simulink library "nort_sysgenlib"  (Simulink 6.5)
undefined symbols (not defined in the file or in its folder): Down, Up
libraries: xbsIndex_r4 x338, nort_sysgenlib x10
(part 1 of 2)
settings Model: Creator=nort  LastModifiedBy=nort

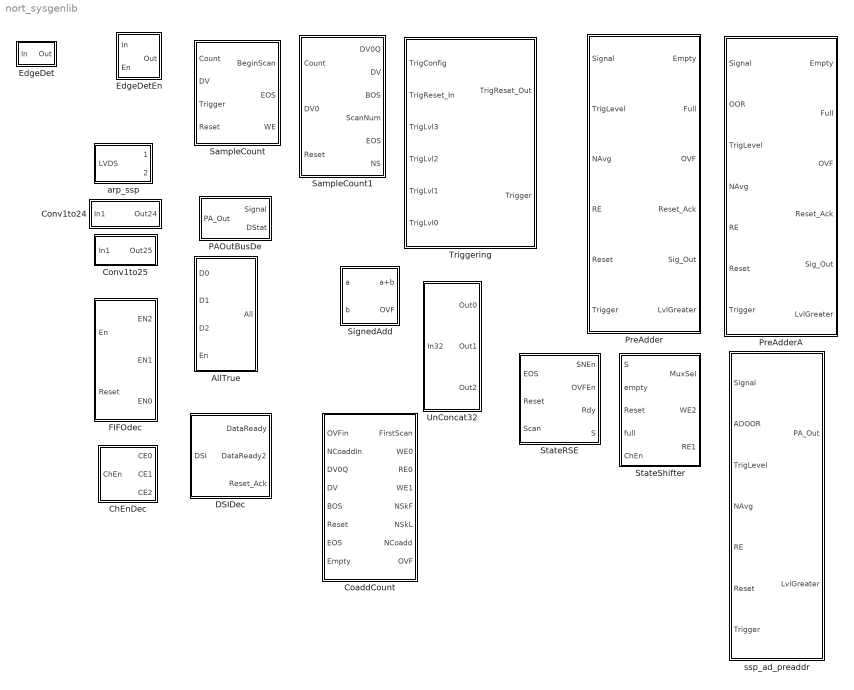
== system nort_sysgenlib ==
  AllTrue : Subsystem
  ChEnDec : Subsystem
  CoaddCount : Subsystem
  Conv1to24 : Subsystem
  Conv1to25 : Subsystem
  DSIDec : Subsystem
  EdgeDet : Subsystem
  EdgeDetEn : Subsystem
  FIFOdec : Subsystem
  PAOutBusDe : Subsystem
  PreAdder : Subsystem
  PreAdderA : Subsystem
  SampleCount : Subsystem
  SampleCount1 : Subsystem
  SignedAdd : Subsystem
  StateRSE : Subsystem
  StateShifter : Subsystem
  Triggering : Subsystem
  UnConcat32 : Subsystem
  arp_ssp : Subsystem
  ssp_ad_preaddr : Subsystem

== system nort_sysgenlib/AllTrue ==
  note: AllTrue: March 7, 2008
  note: Output is true if all
      | the enabled inputs
      | are true.
  D0 : Inport
  D1 : Inport  Port=2
  D2 : Inport  Port=3
  En : Inport  Port=4
  ChEnDec : nort_sysgenlib/ChEnDec  SystemSampleTime=-1
  Inverter : xbsIndex_r4/Inverter  en=off  latency=0  dbl_ovrd=off  block_type=inv
      settings: block_version=9.2.01
  Inverter1 : xbsIndex_r4/Inverter  en=off  latency=0  dbl_ovrd=off  block_type=inv
      settings: block_version=9.2.01
  Inverter2 : xbsIndex_r4/Inverter  en=off  latency=0  dbl_ovrd=off  block_type=inv
      settings: block_version=9.2.01
  Logical1 : xbsIndex_r4/Logical  logical_function=OR  inputs=2  en=off  latency=0  precision=Full  arith_type=Unsigned  n_bits=16  bin_pt=0  align_bp=on  dbl_ovrd=off  block_type=logical
      settings: block_version=9.2.01
  Logical2 : xbsIndex_r4/Logical  logical_function=AND  inputs=3  en=off  latency=0  precision=Full  arith_type=Unsigned  n_bits=16  bin_pt=0  align_bp=on  dbl_ovrd=off  block_type=logical
      settings: block_version=9.2.01
  Logical4 : xbsIndex_r4/Logical  logical_function=OR  inputs=2  en=off  latency=0  precision=Full  arith_type=Unsigned  n_bits=16  bin_pt=0  align_bp=on  dbl_ovrd=off  block_type=logical
      settings: block_version=9.2.01
  Logical6 : xbsIndex_r4/Logical  logical_function=OR  inputs=2  en=off  latency=0  precision=Full  arith_type=Unsigned  n_bits=16  bin_pt=0  align_bp=on  dbl_ovrd=off  block_type=logical
      settings: block_version=9.2.01
  All : Outport
  wires:
  En/1 -> ChEnDec/1
  ChEnDec/3 -> Inverter2/1
  ChEnDec/2 -> Inverter1/1
  ChEnDec/1 -> Inverter/1
  D2/1 -> Logical6/1
  Logical2/1 -> All/1
  D1/1 -> Logical4/1
  D0/1 -> Logical1/1
  Logical6/1 -> Logical2/3
  Logical1/1 -> Logical2/1
  Logical4/1 -> Logical2/2
  Inverter/1 -> Logical1/2
  Inverter1/1 -> Logical4/2
  Inverter2/1 -> Logical6/2

== system nort_sysgenlib/ChEnDec ==
  note: ChEnDec: March 7, 2008
  ChEn : Inport
  ChEnblBit0 : xbsIndex_r4/Slice  nbits=3  boolean_output=on  mode=Lower Bit Location + Width  bit1=0  base1=MSB of Input  bit0=0  base0=LSB of Input  dbl_ovrd=off  block_type=slice
      settings: infoedit="Extracts a given range of bits from each input sample and presents it at the output.  The output type is ordinarily unsigned with binary point at zero, but can be Boolean when the slice is one bit wide.<P><P>Hardware notes: In hardware this block costs nothing."  block_version=8.2
  ChEnblBit1 : xbsIndex_r4/Slice  nbits=3  boolean_output=on  mode=Lower Bit Location + Width  bit1=0  base1=MSB of Input  bit0=1  base0=LSB of Input  dbl_ovrd=off  block_type=slice
      settings: infoedit="Extracts a given range of bits from each input sample and presents it at the output.  The output type is ordinarily unsigned with binary point at zero, but can be Boolean when the slice is one bit wide.<P><P>Hardware notes: In hardware this block costs nothing."  block_version=8.2
  ChEnblBit2 : xbsIndex_r4/Slice  nbits=3  boolean_output=on  mode=Lower Bit Location + Width  bit1=0  base1=MSB of Input  bit0=2  base0=LSB of Input  dbl_ovrd=off  block_type=slice
      settings: infoedit="Extracts a given range of bits from each input sample and presents it at the output.  The output type is ordinarily unsigned with binary point at zero, but can be Boolean when the slice is one bit wide.<P><P>Hardware notes: In hardware this block costs nothing."  block_version=8.2
  CE0 : Outport
  CE1 : Outport  Port=2
  CE2 : Outport  Port=3
  wires:
  ChEnblBit2/1 -> CE2/1
  ChEnblBit1/1 -> CE1/1
  ChEnblBit0/1 -> CE0/1
  ChEn/1 -> ChEnblBit2/1, ChEnblBit1/1, ChEnblBit0/1

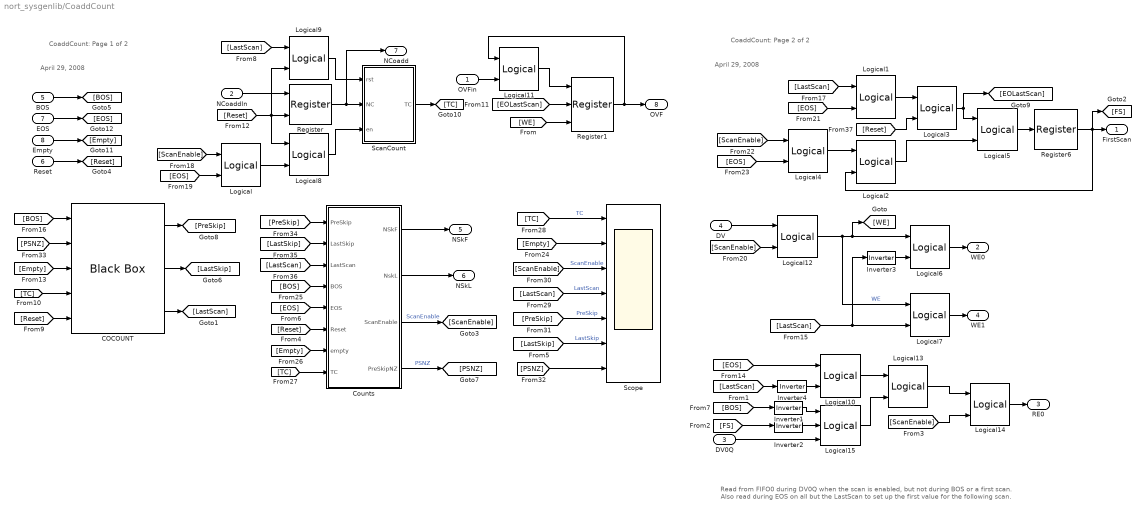
== system nort_sysgenlib/CoaddCount ==
  note: Read from FIFO0 during DV0Q when the scan is enabled, but not during BOS or a first scan.
      | Also read during EOS on all but the LastScan to set up the first value for the following scan.
  note: April 29, 2008
  note: CoaddCount: Page 2 of 2
  note: April 29, 2008
  note: CoaddCount: Page 1 of 2
  OVFin : Inport
  NCoaddIn : Inport  Port=2
  DV0Q : Inport  Port=3
  DV : Inport  Port=4
  BOS : Inport  Port=5
  Reset : Inport  Port=6
  EOS : Inport  Port=7
  Empty : Inport  Port=8
  COCOUNT : xbsIndex_r4/Black Box  init_code=COCOUNT_config  sim_method=ISE Simulator  block_type=blackbox2
      settings: infoedit="Incorporates black box HDL and simulation model into a System Generator design.<P><P>You must supply a Black Box with certain information about the HDL component you would like to bring into System Generator. This information is provided through a Matlab function.<P><P>When \"Simulation mode\" is set to \"Inactive\", you will typically want to provide a separate simulation model by using a Simulation Multiplexer.<P>When \"Simulation mode\" is set to \"External co-simulator\", you must include a ModelSim block in the design."  block_version=9.2.01
  Counts : Subsystem
  Inverter{1..4} (4 alike) : xbsIndex_r4/Inverter  en=off  latency=0  dbl_ovrd=off  block_type=inv
      settings: block_version=9.2.01
  Logical{,1..2,6..7,10,12,14} (8 alike) : xbsIndex_r4/Logical  logical_function=AND  inputs=2  en=off  latency=0  precision=Full  arith_type=Unsigned  n_bits=16  bin_pt=0  align_bp=on  dbl_ovrd=off  block_type=logical
      settings: block_version=9.2.01
  Logical{3,5,8..9,11,13} (6 alike) : xbsIndex_r4/Logical  logical_function=OR  inputs=2  en=off  latency=0  precision=Full  arith_type=Unsigned  n_bits=16  bin_pt=0  align_bp=on  dbl_ovrd=off  block_type=logical
      settings: block_version=9.2.01
  Logical15 : xbsIndex_r4/Logical  logical_function=AND  inputs=3  en=off  latency=0  precision=Full  arith_type=Unsigned  n_bits=16  bin_pt=0  align_bp=on  dbl_ovrd=off  block_type=logical
      settings: block_version=9.2.01
  Logical4 : xbsIndex_r4/Logical  logical_function=NAND  inputs=2  en=off  latency=0  precision=Full  arith_type=Unsigned  n_bits=16  bin_pt=0  align_bp=on  dbl_ovrd=off  block_type=logical
      settings: block_version=9.2.01
  Register : xbsIndex_r4/Register  init=0  rst=off  en=on  dbl_ovrd=off  block_type=register
      settings: block_version=9.2.01
  Register1 : xbsIndex_r4/Register  init=0  rst=on  en=on  dbl_ovrd=off  block_type=register
      settings: block_version=9.2.01
  Register6 : xbsIndex_r4/Register  init=0  rst=off  en=off  dbl_ovrd=off  block_type=register
      settings: block_version=9.2.01
  ScanCount : Subsystem
  Scope : Scope  NumInputPorts=7
      settings: TickLabels=on  TimeRange=5000  YMin=-0.25~-0.25~-0.15~-0.25~-0.25~-0.25~-0.25  YMax=1.25~1.25~1.25~1.25~1.25~1.25~1.25
  FirstScan : Outport
  WE0 : Outport  Port=2
  RE0 : Outport  Port=3
  WE1 : Outport  Port=4
  NSkF : Outport  Port=5
  NSkL : Outport  Port=6
  NCoadd : Outport  Port=7
  OVF : Outport  Port=8
  wires:
  Logical3/1 -> [EOLastScan], Logical5/1
  Logical5/1 -> Register6/1
  Inverter2/1 -> Logical15/2
  Inverter1/1 -> Logical15/1
  [Reset] -> Logical3/2
  [LastScan] -> Counts/3(LastScan)
  [LastSkip] -> Counts/2(LastSkip)
  [PreSkip] -> Counts/1(PreSkip)
  [PSNZ] -> COCOUNT/2
  [PSNZ] -> Scope/7
  [TC] -> Counts/8(TC)
  [Empty] -> Counts/7(empty)
  [BOS] -> Counts/4(BOS)
  COCOUNT/2 -> [LastSkip]
  COCOUNT/3 -> [LastScan]
  [Empty] -> Scope/2
  [ScanEnable] -> Logical14/2
  [EOS] -> Logical4/2
  [ScanEnable] -> Logical4/1
  Logical4/1 -> Logical2/1
  Logical2/1 -> Logical5/2
  Logical1/1 -> Logical3/1
  [EOS] -> Logical1/2
  [LastScan] -> Logical1/1
  [EOS] -> Logical/2
  [ScanEnable] -> Logical/1
  Counts/4(PreSkipNZ) -> [PSNZ]  "PSNZ"
  [BOS] -> COCOUNT/1
  [Empty] -> COCOUNT/3
  [TC] -> COCOUNT/4
  [Reset] -> COCOUNT/5
  [LastScan] -> Logical9/1
  EOS/1 -> [EOS]
  [LastSkip] -> Scope/6  "LastSkip"
  [PreSkip] -> Scope/5  "PreSkip"
  [ScanEnable] -> Scope/3  "ScanEnable"
  [LastScan] -> Scope/4  "LastScan"
  [TC] -> Scope/1  "TC"
  Logical14/1 -> RE0/1
  Logical15/1 -> Logical13/2
  [FS] -> Inverter2/1
  Inverter4/1 -> Logical10/2
  Logical10/1 -> Logical13/1
  DV0Q/1 -> Logical15/3
  Logical13/1 -> Logical14/1
  [LastScan] -> Inverter4/1
  Logical11/1 -> Register1/1
  [WE] -> Register1/3
  Logical12/1 -> Logical7/1, Logical6/1, [WE]  "WE"
  Register1/1 -> Logical11/1, OVF/1
  OVFin/1 -> Logical11/2
  Logical9/1 -> ScanCount/1(rst)
  Logical8/1 -> ScanCount/3(en)
  Logical7/1 -> WE1/1
  Logical6/1 -> WE0/1
  Inverter3/1 -> Logical6/2
  DV/1 -> Logical12/1
  Counts/3(ScanEnable) -> [ScanEnable]  "ScanEnable"
  COCOUNT/1 -> [PreSkip]
  BOS/1 -> [BOS]
  Empty/1 -> [Empty]
  ScanCount/1(TC) -> [TC]
  Register6/1 -> Logical2/2, [FS], FirstScan/1
  Counts/2(NskL) -> NSkL/1
  Counts/1(NSkF) -> NSkF/1
  Register/1 -> NCoadd/1, ScanCount/2(NC)
  NCoaddIn/1 -> Register/1
  Reset/1 -> [Reset]
  [Reset] -> Counts/6(Reset)
  [EOS] -> Counts/5(EOS)
  [BOS] -> Inverter1/1
  [EOLastScan] -> Register1/2
  [Reset] -> Logical8/1, Register/2, Logical9/2
  Logical/1 -> Logical8/2
  [EOS] -> Logical10/1
  [LastScan] -> Logical7/2, Inverter3/1
  [ScanEnable] -> Logical12/2

== system nort_sysgenlib/Conv1to24 ==
  In1 : Inport
  To24Bits : xbsIndex_r4/Convert  arith_type="Signed  (2's comp)"  n_bits=24  bin_pt=0  quantization=Truncate  overflow=Wrap  latency=0  dbl_ovrd=off  pipeline=off  block_type=convert
      settings: block_version=9.2.01
  ToSigned : xbsIndex_r4/Convert  arith_type="Signed  (2's comp)"  n_bits=1  bin_pt=0  quantization=Truncate  overflow=Wrap  latency=0  dbl_ovrd=off  pipeline=off  block_type=convert
      settings: block_version=9.2.01
  Out24 : Outport
  wires:
  In1/1 -> ToSigned/1
  ToSigned/1 -> To24Bits/1
  To24Bits/1 -> Out24/1

== system nort_sysgenlib/Conv1to25 ==
  In1 : Inport
  To25Bits : xbsIndex_r4/Convert  arith_type="Signed  (2's comp)"  n_bits=25  bin_pt=0  quantization=Truncate  overflow=Wrap  latency=0  dbl_ovrd=off  pipeline=off  block_type=convert
      settings: block_version=9.2.01
  ToSigned : xbsIndex_r4/Convert  arith_type="Signed  (2's comp)"  n_bits=1  bin_pt=0  quantization=Truncate  overflow=Wrap  latency=0  dbl_ovrd=off  pipeline=off  block_type=convert
      settings: block_version=9.2.01
  Out25 : Outport
  wires:
  In1/1 -> ToSigned/1
  ToSigned/1 -> To25Bits/1
  To25Bits/1 -> Out25/1

== system nort_sysgenlib/DSIDec ==
  note: DSIDec: April 29, 2008
  DSI : Inport
  Empty_Bit2 : xbsIndex_r4/Slice  nbits=1  boolean_output=on  mode=Lower Bit Location + Width  bit1=0  base1=MSB of Input  bit0=2  base0=LSB of Input  dbl_ovrd=off  block_type=slice
      settings: infoedit="Extracts a given range of bits from each input sample and presents it at the output.  The output type is ordinarily unsigned with binary point at zero, but can be Boolean when the slice is one bit wide.<P><P>Hardware notes: In hardware this block costs nothing."  block_version=9.2.01
  Full_Bit1 : xbsIndex_r4/Slice  nbits=1  boolean_output=on  mode=Lower Bit Location + Width  bit1=0  base1=MSB of Input  bit0=1  base0=LSB of Input  dbl_ovrd=off  block_type=slice
      settings: infoedit="Extracts a given range of bits from each input sample and presents it at the output.  The output type is ordinarily unsigned with binary point at zero, but can be Boolean when the slice is one bit wide.<P><P>Hardware notes: In hardware this block costs nothing."  block_version=9.2.01
  Inverter2 : xbsIndex_r4/Inverter  en=off  latency=0  dbl_ovrd=off  block_type=inv
      settings: block_version=9.2.01
  RAck_Bit0 : xbsIndex_r4/Slice  nbits=1  boolean_output=on  mode=Lower Bit Location + Width  bit1=0  base1=MSB of Input  bit0=0  base0=LSB of Input  dbl_ovrd=off  block_type=slice
      settings: infoedit="Extracts a given range of bits from each input sample and presents it at the output.  The output type is ordinarily unsigned with binary point at zero, but can be Boolean when the slice is one bit wide.<P><P>Hardware notes: In hardware this block costs nothing."  block_version=9.2.01
  DataReady : Outport
  DataReady2 : Outport  Port=2
  Reset_Ack : Outport  Port=3
  wires:
  RAck_Bit0/1 -> Reset_Ack/1
  Full_Bit1/1 -> DataReady2/1
  Inverter2/1 -> DataReady/1
  Empty_Bit2/1 -> Inverter2/1
  DSI/1 -> RAck_Bit0/1, Full_Bit1/1, Empty_Bit2/1

== system nort_sysgenlib/EdgeDet ==
  note: Simple Edge Detector
  In : Inport
  Delay : xbsIndex_r4/Delay  en=off  latency=1  dbl_ovrd=off  reg_retiming=off  block_type=delay
      settings: block_version=9.1.01
  Delay1 : xbsIndex_r4/Delay  en=off  latency=1  dbl_ovrd=off  reg_retiming=off  block_type=delay
      settings: block_version=9.1.01
  Inverter1 : xbsIndex_r4/Inverter  en=off  latency=0  dbl_ovrd=off  block_type=inv
      settings: block_version=9.1.01
  Logical3 : xbsIndex_r4/Logical  logical_function=AND  inputs=2  en=off  latency=0  precision=Full  arith_type=Unsigned  n_bits=16  bin_pt=0  align_bp=on  dbl_ovrd=off  block_type=logical
      settings: block_version=9.1.01
  Out : Outport
  wires:
  Delay1/1 -> Delay/1, Logical3/2
  Logical3/1 -> Out/1
  Inverter1/1 -> Logical3/1
  Delay/1 -> Inverter1/1
  In/1 -> Delay1/1

== system nort_sysgenlib/EdgeDetEn ==
  note: Edge Detection with Enable
  In : Inport
  En : Inport  Port=2
  Delay : xbsIndex_r4/Delay  en=off  latency=1  dbl_ovrd=off  reg_retiming=off  block_type=delay
      settings: block_version=9.1.01
  Delay1 : xbsIndex_r4/Delay  en=on  latency=1  dbl_ovrd=off  reg_retiming=off  block_type=delay
      settings: block_version=9.1.01
  Inverter1 : xbsIndex_r4/Inverter  en=off  latency=0  dbl_ovrd=off  block_type=inv
      settings: block_version=9.1.01
  Logical3 : xbsIndex_r4/Logical  logical_function=AND  inputs=2  en=off  latency=0  precision=Full  arith_type=Unsigned  n_bits=16  bin_pt=0  align_bp=on  dbl_ovrd=off  block_type=logical
      settings: block_version=9.1.01
  Out : Outport
  wires:
  En/1 -> Delay1/2
  In/1 -> Delay1/1
  Delay1/1 -> Delay/1, Logical3/2
  Logical3/1 -> Out/1
  Inverter1/1 -> Logical3/1
  Delay/1 -> Inverter1/1

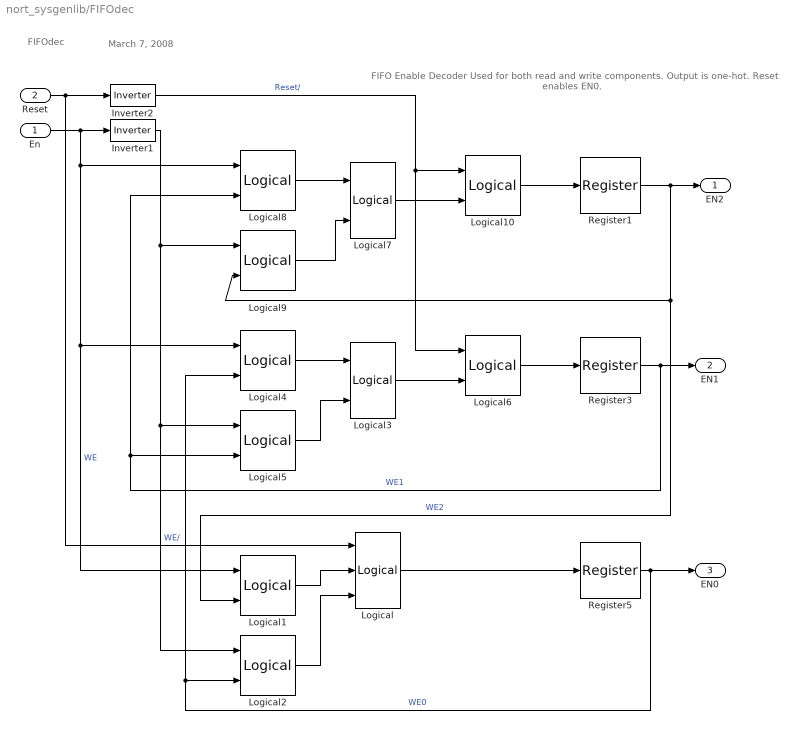
== system nort_sysgenlib/FIFOdec ==
  note: FIFO Enable Decoder
      | Used for both read and write components.
      | Output is one-hot. Reset enables EN0.
  note: March 7, 2008
  note: FIFOdec
  En : Inport
  Reset : Inport  Port=2
  Inverter1 : xbsIndex_r4/Inverter  en=off  latency=0  dbl_ovrd=off  block_type=inv
      settings: block_version=9.2.01
  Inverter2 : xbsIndex_r4/Inverter  en=off  latency=0  dbl_ovrd=off  block_type=inv
      settings: block_version=9.2.01
  Logical : xbsIndex_r4/Logical  logical_function=OR  inputs=3  en=off  latency=0  precision=Full  arith_type=Unsigned  n_bits=16  bin_pt=0  align_bp=on  dbl_ovrd=off  block_type=logical
      settings: block_version=9.2.01
  Logical{1..2,4..6,8..10} (8 alike) : xbsIndex_r4/Logical  logical_function=AND  inputs=2  en=off  latency=0  precision=Full  arith_type=Unsigned  n_bits=16  bin_pt=0  align_bp=on  dbl_ovrd=off  block_type=logical
      settings: block_version=9.2.01
  Logical3 : xbsIndex_r4/Logical  logical_function=OR  inputs=2  en=off  latency=0  precision=Full  arith_type=Unsigned  n_bits=16  bin_pt=0  align_bp=on  dbl_ovrd=off  block_type=logical
      settings: block_version=9.2.01
  Logical7 : xbsIndex_r4/Logical  logical_function=OR  inputs=2  en=off  latency=0  precision=Full  arith_type=Unsigned  n_bits=16  bin_pt=0  align_bp=on  dbl_ovrd=off  block_type=logical
      settings: block_version=9.2.01
  Register1 : xbsIndex_r4/Register  init=0  rst=off  en=off  dbl_ovrd=off  block_type=register
      settings: block_version=9.2.01
  Register3 : xbsIndex_r4/Register  init=0  rst=off  en=off  dbl_ovrd=off  block_type=register
      settings: block_version=9.2.01
  Register5 : xbsIndex_r4/Register  init=0  rst=off  en=off  dbl_ovrd=off  block_type=register
      settings: block_version=9.2.01
  EN2 : Outport
  EN1 : Outport  Port=2
  EN0 : Outport  Port=3
  wires:
  Logical8/1 -> Logical7/1
  Inverter2/1 -> Logical10/1, Logical6/1  "Reset/"
  Logical10/1 -> Register1/1
  Logical7/1 -> Logical10/2
  Logical9/1 -> Logical7/2
  Logical6/1 -> Register3/1
  Logical3/1 -> Logical6/2
  Logical4/1 -> Logical3/1
  Logical5/1 -> Logical3/2
  Logical1/1 -> Logical/2
  Logical2/1 -> Logical/3
  Inverter1/1 -> Logical9/1, Logical5/1, Logical2/1  "WE/"
  En/1 -> Logical8/1, Logical4/1, Logical1/1, Inverter1/1  "WE"
  Reset/1 -> Inverter2/1, Logical/1
  Logical/1 -> Register5/1
  Register5/1 -> Logical4/2, Logical2/2, EN0/1  "WE0"
  Register3/1 -> Logical8/2, Logical5/2, EN1/1  "WE1"
  Register1/1 -> Logical9/2, Logical1/2, EN2/1  "WE2"

== system nort_sysgenlib/PAOutBusDe ==
  note: PAOutBusDecode: April 29, 2008
  PA_Out : Inport
  DS_Bot3 : xbsIndex_r4/Slice  nbits=3  boolean_output=off  mode=Lower Bit Location + Width  bit1=0  base1=MSB of Input  bit0=0  base0=LSB of Input  dbl_ovrd=off  block_type=slice
      settings: infoedit="Extracts a given range of bits from each input sample and presents it at the output.  The output type is ordinarily unsigned with binary point at zero, but can be Boolean when the slice is one bit wide.<P><P>Hardware notes: In hardware this block costs nothing."  block_version=9.2.01
  Sig_Top26 : xbsIndex_r4/Slice  nbits=26  boolean_output=off  mode=Lower Bit Location + Width  bit1=0  base1=MSB of Input  bit0=3  base0=LSB of Input  dbl_ovrd=off  block_type=slice
      settings: infoedit="Extracts a given range of bits from each input sample and presents it at the output.  The output type is ordinarily unsigned with binary point at zero, but can be Boolean when the slice is one bit wide.<P><P>Hardware notes: In hardware this block costs nothing."  block_version=9.2.01
  Signal : Outport
  DStat : Outport  Port=2
  wires:
  DS_Bot3/1 -> DStat/1
  Sig_Top26/1 -> Signal/1
  PA_Out/1 -> Sig_Top26/1, DS_Bot3/1

== system nort_sysgenlib/PreAdder ==
  note: February 29, 2008
  note: ssp_ad_preaddr V2.00a
  Signal : Inport
  TrigLevel : Inport  Port=2
  NAvg : Inport  Port=3
  RE : Inport  Port=4
  Reset : Inport  Port=5
  Trigger : Inport  Port=6
  AddSub : xbsIndex_r4/AddSub  mode=Addition  use_carryin=off  use_carryout=off  en=off  latency=0  precision=User Defined  arith_type="Signed  (2's comp)"  n_bits=24  bin_pt=0  quantization=Truncate  overflow=Saturate  dbl_ovrd=off  use_behavioral_HDL=off  pipelined=off  use_rpm=on  block_type=addsub
      settings: block_version=9.1.01
  Count : Subsystem
  FIFO : Subsystem
  Logical : xbsIndex_r4/Logical  logical_function=OR  inputs=2  en=off  latency=0  precision=Full  arith_type=Unsigned  n_bits=16  bin_pt=0  align_bp=on  dbl_ovrd=off  block_type=logical
      settings: block_version=9.2.01
  Register : xbsIndex_r4/Register  init=0  rst=on  en=off  dbl_ovrd=off  block_type=register
      settings: block_version=9.1.01
  Relational : xbsIndex_r4/Relational  mode=a>b  en=off  latency=0  dbl_ovrd=off  block_type=relational
      settings: block_version=9.2.01
  State : Subsystem
  Empty : Outport
  Full : Outport  Port=2
  OVF : Outport  Port=3
  Reset_Ack : Outport  Port=4
  Sig_Out : Outport  Port=5
  LvlGreater : Outport  Port=6
  wires:
  FIFO/3(Full) -> Full/1  "Full"
  State/1(Inactive) -> Logical/2, Count/2(Reset)
  FIFO/4(OVF) -> OVF/1  "OVF"
  Trigger/1 -> State/2(Trigger)
  FIFO/2(Empty) -> Empty/1  "Empty"
  Reset/1 -> State/1(ResIn)
  NAvg/1 -> Count/1(NA)
  TrigLevel/1 -> Relational/2
  Relational/1 -> LvlGreater/1
  RE/1 -> FIFO/3(RE)
  Count/1(NewData) -> FIFO/2(WE), Logical/1  "NewData"
  Logical/1 -> Register/2
  State/2(Reset) -> Reset_Ack/1, FIFO/4(Reset)
  FIFO/1(Dout) -> Sig_Out/1  "Sig_Out"
  Signal/1 -> AddSub/2, Relational/1
  Register/1 -> AddSub/1
  AddSub/1 -> FIFO/1(Din), Register/1

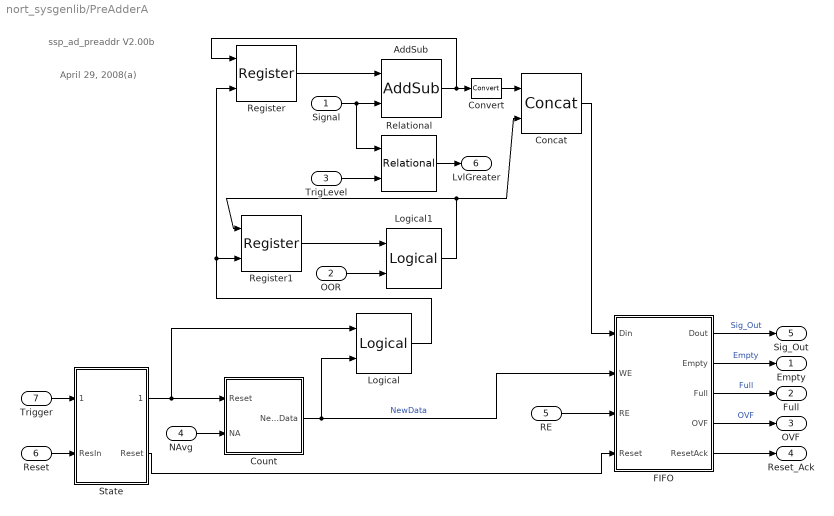
== system nort_sysgenlib/PreAdderA ==
  note: April 29, 2008(a)
  note: ssp_ad_preaddr V2.00b
  Signal : Inport
  OOR : Inport  Port=2
  TrigLevel : Inport  Port=3
  NAvg : Inport  Port=4
  RE : Inport  Port=5
  Reset : Inport  Port=6
  Trigger : Inport  Port=7
  AddSub : xbsIndex_r4/AddSub  mode=Addition  use_carryin=off  use_carryout=off  en=off  latency=0  precision=User Defined  arith_type="Signed  (2's comp)"  n_bits=24  bin_pt=0  quantization=Truncate  overflow=Saturate  dbl_ovrd=off  use_behavioral_HDL=off  pipelined=off  use_rpm=on  block_type=addsub
      settings: block_version=9.1.01
  Concat : xbsIndex_r4/Concat  num_inputs=2  dbl_ovrd=off  block_type=concat
      settings: block_version=9.2.01
  Convert : xbsIndex_r4/Convert  arith_type=Unsigned  n_bits=24  bin_pt=0  quantization=Truncate  overflow=Wrap  latency=0  dbl_ovrd=off  pipeline=off  block_type=convert
      settings: block_version=9.2.01
  Count : Subsystem
  FIFO : Subsystem
  Logical : xbsIndex_r4/Logical  logical_function=OR  inputs=2  en=off  latency=0  precision=Full  arith_type=Unsigned  n_bits=16  bin_pt=0  align_bp=on  dbl_ovrd=off  block_type=logical
      settings: block_version=9.2.01
  Logical1 : xbsIndex_r4/Logical  logical_function=OR  inputs=2  en=off  latency=0  precision=Full  arith_type=Unsigned  n_bits=16  bin_pt=0  align_bp=on  dbl_ovrd=off  block_type=logical
      settings: block_version=9.2.01
  Register : xbsIndex_r4/Register  init=0  rst=on  en=off  dbl_ovrd=off  block_type=register
      settings: block_version=9.1.01
  Register1 : xbsIndex_r4/Register  init=0  rst=on  en=off  dbl_ovrd=off  block_type=register
      settings: block_version=9.1.01
  Relational : xbsIndex_r4/Relational  mode=a>b  en=off  latency=0  dbl_ovrd=off  block_type=relational
      settings: block_version=9.2.01
  State : Subsystem
  Empty : Outport
  Full : Outport  Port=2
  OVF : Outport  Port=3
  Reset_Ack : Outport  Port=4
  Sig_Out : Outport  Port=5
  LvlGreater : Outport  Port=6
  wires:
  Logical/1 -> Register1/2, Register/2
  FIFO/5(ResetAck) -> Reset_Ack/1
  Convert/1 -> Concat/1
  FIFO/3(Full) -> Full/1  "Full"
  State/1(Inactive) -> Logical/1, Count/1(Reset)
  FIFO/4(OVF) -> OVF/1  "OVF"
  Trigger/1 -> State/1(Trigger)
  FIFO/2(Empty) -> Empty/1  "Empty"
  Reset/1 -> State/2(ResIn)
  NAvg/1 -> Count/2(NA)
  TrigLevel/1 -> Relational/2
  Relational/1 -> LvlGreater/1
  RE/1 -> FIFO/3(RE)
  Count/1(NewData) -> Logical/2, FIFO/2(WE)  "NewData"
  State/2(Reset) -> FIFO/4(Reset)
  FIFO/1(Dout) -> Sig_Out/1  "Sig_Out"
  Signal/1 -> AddSub/2, Relational/1
  Register/1 -> AddSub/1
  AddSub/1 -> Convert/1, Register/1
  Logical1/1 -> Concat/2, Register1/1
  Register1/1 -> Logical1/1
  OOR/1 -> Logical1/2
  Concat/1 -> FIFO/1(Din)

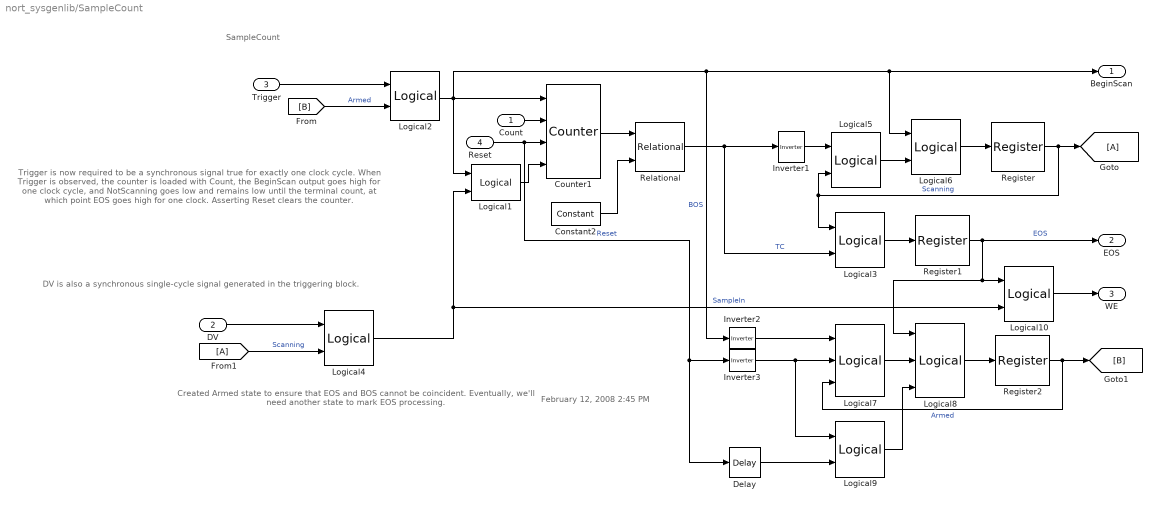
== system nort_sysgenlib/SampleCount ==
  note: Trigger is now required to be a
      | synchronous signal true for exactly
      | one clock cycle. When Trigger
      | is observed, the counter is loaded
      | with Count, the BeginScan output goes
      | high for one clock cycle, and
      | NotScanning goes low and remains low
      | until the terminal count, at which point
      | EOS goes high for one clock.
      | Asserting Reset clears the counter.
  note: February 12, 2008 2:45 PM
  note: DV is also a synchronous single-cycle signal
      | generated in the triggering block.
  note: SampleCount
  note: Created Armed state to ensure that EOS and BOS cannot be coincident.
      | Eventually, we'll need another state to mark EOS processing.
  Count : Inport
  DV : Inport  Port=2
  Trigger : Inport  Port=3
  Reset : Inport  Port=4
  Constant2 : xbsIndex_r4/Constant  arith_type=Unsigned  const=0  n_bits=11  bin_pt=0  explicit_period=off  period=1  equ=P=C  opselect=C  inp2=PCIN>>17  opr=+  inp1=P  carry=CIN  dbl_ovrd=off  block_type=constant
      settings: block_version=8.2
  Counter1 : xbsIndex_r4/Counter  cnt_type=Free Running  cnt_to=Inf  operation=Down  start_count=0  cnt_by_val=1  arith_type=Unsigned  n_bits=12  bin_pt=0  load_pin=on  rst=on  en=on  explicit_period=off  period=1  dbl_ovrd=off  use_behavioral_HDL=off  use_rpm=off  block_type=counter
      settings: block_version=8.2
  Delay : xbsIndex_r4/Delay  en=off  latency=1  dbl_ovrd=off  reg_retiming=off  block_type=delay
      settings: block_version=9.2.01
  Inverter1 : xbsIndex_r4/Inverter  en=off  latency=0  dbl_ovrd=off  block_type=inv
      settings: block_version=8.2
  Inverter2 : xbsIndex_r4/Inverter  en=off  latency=0  dbl_ovrd=off  block_type=inv
      settings: block_version=8.2
  Inverter3 : xbsIndex_r4/Inverter  en=off  latency=0  dbl_ovrd=off  block_type=inv
      settings: block_version=8.2
  Logical1 : xbsIndex_r4/Logical  logical_function=OR  inputs=2  en=off  latency=0  precision=Full  arith_type=Unsigned  n_bits=16  bin_pt=0  align_bp=on  dbl_ovrd=off  block_type=logical
      settings: block_version=8.2
  Logical10 : xbsIndex_r4/Logical  logical_function=OR  inputs=2  en=off  latency=0  precision=Full  arith_type=Unsigned  n_bits=1  bin_pt=0  align_bp=off  dbl_ovrd=off  block_type=logical
      settings: block_version=8.2
  Logical2 : xbsIndex_r4/Logical  logical_function=AND  inputs=2  en=off  latency=0  precision=Full  arith_type=Unsigned  n_bits=16  bin_pt=0  align_bp=on  dbl_ovrd=off  block_type=logical
      settings: block_version=8.2
  Logical{3..5,9} (4 alike) : xbsIndex_r4/Logical  logical_function=AND  inputs=2  en=off  latency=0  precision=Full  arith_type=Unsigned  n_bits=1  bin_pt=0  align_bp=off  dbl_ovrd=off  block_type=logical
      settings: block_version=8.2
  Logical6 : xbsIndex_r4/Logical  logical_function=OR  inputs=2  en=off  latency=0  precision=Full  arith_type=Unsigned  n_bits=1  bin_pt=0  align_bp=off  dbl_ovrd=off  block_type=logical
      settings: block_version=8.2
  Logical7 : xbsIndex_r4/Logical  logical_function=AND  inputs=3  en=off  latency=0  precision=Full  arith_type=Unsigned  n_bits=1  bin_pt=0  align_bp=off  dbl_ovrd=off  block_type=logical
      settings: block_version=8.2
  Logical8 : xbsIndex_r4/Logical  logical_function=OR  inputs=3  en=off  latency=0  precision=Full  arith_type=Unsigned  n_bits=1  bin_pt=0  align_bp=off  dbl_ovrd=off  block_type=logical
      settings: block_version=8.2
  Register : xbsIndex_r4/Register  init=0  rst=off  en=off  dbl_ovrd=off  block_type=register
      settings: block_version=9.2.01
  Register1 : xbsIndex_r4/Register  init=0  rst=off  en=off  dbl_ovrd=off  block_type=register
      settings: block_version=9.2.01
  Register2 : xbsIndex_r4/Register  init=0  rst=off  en=off  dbl_ovrd=off  block_type=register
      settings: block_version=9.2.01
  Relational : xbsIndex_r4/Relational  mode=a=b  en=off  latency=0  dbl_ovrd=off  block_type=relational
      settings: block_version=8.2
  BeginScan : Outport
  EOS : Outport  Port=2
  WE : Outport  Port=3
  wires:
  Counter1/1 -> Relational/1
  Logical1/1 -> Counter1/4
  Constant2/1 -> Relational/2
  Logical2/1 -> Counter1/1, Logical1/1, BeginScan/1, Logical6/1, Inverter2/1  "BOS"
  Count/1 -> Counter1/2
  Trigger/1 -> Logical2/1
  Reset/1 -> Counter1/3, Delay/1, Inverter3/1  "Reset"
  Logical4/1 -> Logical10/2, Logical1/2  "SampleIn"
  [A] -> Logical4/2  "Scanning"
  DV/1 -> Logical4/1
  Logical5/1 -> Logical6/2
  Logical6/1 -> Register/1
  Inverter1/1 -> Logical5/1
  Relational/1 -> Logical3/2, Inverter1/1  "TC"
  Register/1 -> Logical5/2, Logical3/1, [A]  "Scanning"
  Logical3/1 -> Register1/1
  Register1/1 -> EOS/1, Logical8/1, Logical10/1  "EOS"
  Inverter2/1 -> Logical7/1
  Logical8/1 -> Register2/1
  Logical7/1 -> Logical8/2
  Register2/1 -> Logical7/3, [B]  "Armed"
  [B] -> Logical2/2  "Armed"
  Inverter3/1 -> Logical7/2, Logical9/1
  Delay/1 -> Logical9/2
  Logical9/1 -> Logical8/3
  Logical10/1 -> WE/1

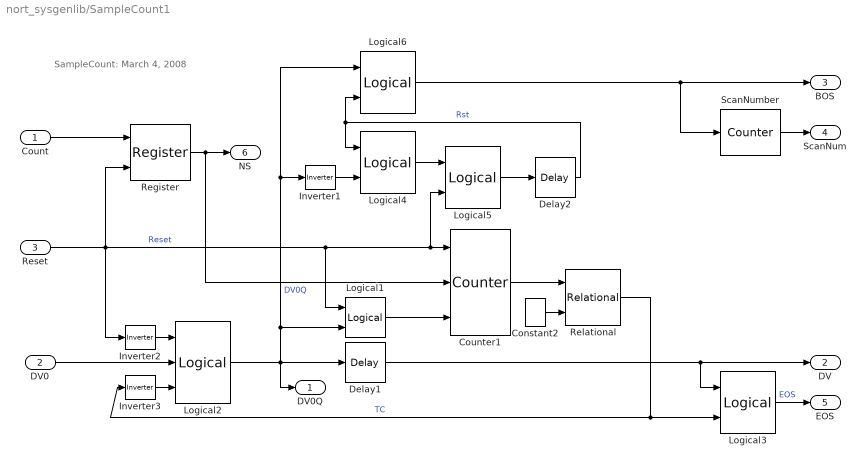
== system nort_sysgenlib/SampleCount1 ==
  note: SampleCount: March 4, 2008
  Count : Inport
  DV0 : Inport  Port=2
  Reset : Inport  Port=3
  Constant2 : xbsIndex_r4/Constant  arith_type=Unsigned  const=0  n_bits=11  bin_pt=0  explicit_period=off  period=1  equ=P=C  opselect=C  inp2=PCIN>>17  opr=+  inp1=P  carry=CIN  dbl_ovrd=off  block_type=constant
      settings: block_version=8.2
  Counter1 : xbsIndex_r4/Counter  cnt_type=Free Running  cnt_to=Inf  operation=Down  start_count=0  cnt_by_val=1  arith_type=Unsigned  n_bits=12  bin_pt=0  load_pin=on  rst=off  en=on  explicit_period=off  period=1  dbl_ovrd=off  use_behavioral_HDL=off  use_rpm=off  block_type=counter
      settings: block_version=8.2
  Delay1 : xbsIndex_r4/Delay  en=off  latency=1  dbl_ovrd=off  reg_retiming=off  block_type=delay
      settings: block_version=9.2.01
  Delay2 : xbsIndex_r4/Delay  en=off  latency=1  dbl_ovrd=off  reg_retiming=off  block_type=delay
      settings: block_version=9.2.01
  Inverter1 : xbsIndex_r4/Inverter  en=off  latency=0  dbl_ovrd=off  block_type=inv
      settings: block_version=8.2
  Inverter2 : xbsIndex_r4/Inverter  en=off  latency=0  dbl_ovrd=off  block_type=inv
      settings: block_version=8.2
  Inverter3 : xbsIndex_r4/Inverter  en=off  latency=0  dbl_ovrd=off  block_type=inv
      settings: block_version=8.2
  Logical1 : xbsIndex_r4/Logical  logical_function=OR  inputs=2  en=off  latency=0  precision=Full  arith_type=Unsigned  n_bits=16  bin_pt=0  align_bp=on  dbl_ovrd=off  block_type=logical
      settings: block_version=8.2
  Logical2 : xbsIndex_r4/Logical  logical_function=AND  inputs=3  en=off  latency=0  precision=Full  arith_type=Unsigned  n_bits=1  bin_pt=0  align_bp=off  dbl_ovrd=off  block_type=logical
      settings: block_version=8.2
  Logical3 : xbsIndex_r4/Logical  logical_function=AND  inputs=2  en=off  latency=0  precision=Full  arith_type=Unsigned  n_bits=1  bin_pt=0  align_bp=off  dbl_ovrd=off  block_type=logical
      settings: block_version=8.2
  Logical4 : xbsIndex_r4/Logical  logical_function=AND  inputs=2  en=off  latency=0  precision=Full  arith_type=Unsigned  n_bits=1  bin_pt=0  align_bp=off  dbl_ovrd=off  block_type=logical
      settings: block_version=8.2
  Logical5 : xbsIndex_r4/Logical  logical_function=OR  inputs=2  en=off  latency=0  precision=Full  arith_type=Unsigned  n_bits=1  bin_pt=0  align_bp=off  dbl_ovrd=off  block_type=logical
      settings: block_version=8.2
  Logical6 : xbsIndex_r4/Logical  logical_function=AND  inputs=2  en=off  latency=0  precision=Full  arith_type=Unsigned  n_bits=1  bin_pt=0  align_bp=off  dbl_ovrd=off  block_type=logical
      settings: block_version=8.2
  Register : xbsIndex_r4/Register  init=0  rst=off  en=on  dbl_ovrd=off  block_type=register
      settings: block_version=9.2.01
  Relational : xbsIndex_r4/Relational  mode=a=b  en=off  latency=0  dbl_ovrd=off  block_type=relational
      settings: block_version=8.2
  ScanNumber : xbsIndex_r4/Counter  cnt_type=Free Running  cnt_to=Inf  operation=Up  start_count=0  cnt_by_val=1  arith_type=Unsigned  n_bits=32  bin_pt=0  load_pin=off  rst=off  en=on  explicit_period=off  period=1  dbl_ovrd=off  use_behavioral_HDL=off  use_rpm=off  block_type=counter
      settings: block_version=8.2
  DV0Q : Outport
  DV : Outport  Port=2
  BOS : Outport  Port=3
  ScanNum : Outport  Port=4
  EOS : Outport  Port=5
  NS : Outport  Port=6
  wires:
  Logical3/1 -> EOS/1  "EOS"
  Relational/1 -> Logical3/2, Inverter3/1  "TC"
  Reset/1 -> Logical1/1, Counter1/1, Logical5/2, Inverter2/1, Register/2  "Reset"
  Constant2/1 -> Relational/2
  Counter1/1 -> Relational/1
  ScanNumber/1 -> ScanNum/1
  Logical1/1 -> Counter1/3
  DV0/1 -> Logical2/2
  Inverter2/1 -> Logical2/1
  Inverter3/1 -> Logical2/3
  Logical2/1 -> Delay1/1, Logical1/2, Inverter1/1, Logical6/1, DV0Q/1  "DV0Q"
  Delay1/1 -> DV/1, Logical3/1
  Logical4/1 -> Logical5/1
  Inverter1/1 -> Logical4/2
  Logical5/1 -> Delay2/1
  Delay2/1 -> Logical4/1, Logical6/2  "Rst"
  Logical6/1 -> BOS/1, ScanNumber/1
  Count/1 -> Register/1
  Register/1 -> NS/1, Counter1/2

== system nort_sysgenlib/SignedAdd ==
  note: SignedAdd with Overflow: April 20, 2008
  a : Inport
  b : Inport  Port=2
  AddSub : xbsIndex_r4/AddSub  mode=Addition  use_carryin=off  use_carryout=off  en=off  latency=0  precision=User Defined  arith_type="Signed  (2's comp)"  n_bits=32  bin_pt=0  quantization=Truncate  overflow=Wrap  dbl_ovrd=off  use_behavioral_HDL=off  pipelined=off  use_rpm=on  block_type=addsub
      settings: block_version=9.2.01
  Convert : xbsIndex_r4/Convert  arith_type=Unsigned  n_bits=32  bin_pt=0  quantization=Truncate  overflow=Wrap  latency=0  dbl_ovrd=off  pipeline=off  block_type=convert
      settings: block_version=9.2.01
  Logical : xbsIndex_r4/Logical  logical_function=XNOR  inputs=2  en=off  latency=0  precision=Full  arith_type=Unsigned  n_bits=16  bin_pt=0  align_bp=on  dbl_ovrd=off  block_type=logical
      settings: block_version=9.2.01
  Logical1 : xbsIndex_r4/Logical  logical_function=XOR  inputs=2  en=off  latency=0  precision=Full  arith_type=Unsigned  n_bits=16  bin_pt=0  align_bp=on  dbl_ovrd=off  block_type=logical
      settings: block_version=9.2.01
  Logical2 : xbsIndex_r4/Logical  logical_function=AND  inputs=2  en=off  latency=0  precision=Full  arith_type=Unsigned  n_bits=16  bin_pt=0  align_bp=on  dbl_ovrd=off  block_type=logical
      settings: block_version=9.2.01
  MSBa : xbsIndex_r4/Slice  nbits=1  boolean_output=on  mode=Upper Bit Location + Width  bit1=0  base1=MSB of Input  bit0=0  base0=LSB of Input  dbl_ovrd=off  block_type=slice
      settings: infoedit="Extracts a given range of bits from each input sample and presents it at the output.  The output type is ordinarily unsigned with binary point at zero, but can be Boolean when the slice is one bit wide.<P><P>Hardware notes: In hardware this block costs nothing."  block_version=9.2.01
  MSBb : xbsIndex_r4/Slice  nbits=1  boolean_output=on  mode=Upper Bit Location + Width  bit1=0  base1=MSB of Input  bit0=0  base0=LSB of Input  dbl_ovrd=off  block_type=slice
      settings: infoedit="Extracts a given range of bits from each input sample and presents it at the output.  The output type is ordinarily unsigned with binary point at zero, but can be Boolean when the slice is one bit wide.<P><P>Hardware notes: In hardware this block costs nothing."  block_version=9.2.01
  MSBsum : xbsIndex_r4/Slice  nbits=1  boolean_output=on  mode=Upper Bit Location + Width  bit1=0  base1=MSB of Input  bit0=0  base0=LSB of Input  dbl_ovrd=off  block_type=slice
      settings: infoedit="Extracts a given range of bits from each input sample and presents it at the output.  The output type is ordinarily unsigned with binary point at zero, but can be Boolean when the slice is one bit wide.<P><P>Hardware notes: In hardware this block costs nothing."  block_version=9.2.01
  a+b : Outport
  OVF : Outport  Port=2
  wires:
  Logical2/1 -> OVF/1
  Convert/1 -> a+b/1
  Logical1/1 -> Logical2/1
  MSBsum/1 -> Logical1/1
  Logical/1 -> Logical2/2
  MSBb/1 -> Logical/2
  MSBa/1 -> Logical1/2, Logical/1
  b/1 -> MSBb/1, AddSub/2
  AddSub/1 -> Convert/1, MSBsum/1
  a/1 -> MSBa/1, AddSub/1

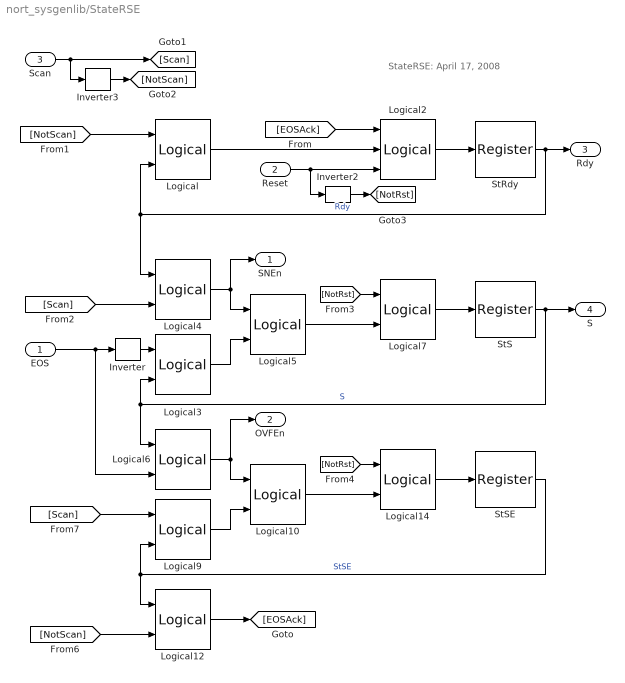
== system nort_sysgenlib/StateRSE ==
  note: StateRSE: April 17, 2008
  EOS : Inport
  Reset : Inport  Port=2
  Scan : Inport  Port=3
  Inverter : xbsIndex_r4/Inverter  en=off  latency=0  dbl_ovrd=off  block_type=inv
      settings: block_version=9.2.01
  Inverter2 : xbsIndex_r4/Inverter  en=off  latency=0  dbl_ovrd=off  block_type=inv
      settings: block_version=9.2.01
  Inverter3 : xbsIndex_r4/Inverter  en=off  latency=0  dbl_ovrd=off  block_type=inv
      settings: block_version=9.2.01
  Logical{,3..4,6..7,9,12,14} (8 alike) : xbsIndex_r4/Logical  logical_function=AND  inputs=2  en=off  latency=0  precision=Full  arith_type=Unsigned  n_bits=16  bin_pt=0  align_bp=on  dbl_ovrd=off  block_type=logical
      settings: block_version=9.2.01
  Logical10 : xbsIndex_r4/Logical  logical_function=OR  inputs=2  en=off  latency=0  precision=Full  arith_type=Unsigned  n_bits=16  bin_pt=0  align_bp=on  dbl_ovrd=off  block_type=logical
      settings: block_version=9.2.01
  Logical2 : xbsIndex_r4/Logical  logical_function=OR  inputs=3  en=off  latency=0  precision=Full  arith_type=Unsigned  n_bits=16  bin_pt=0  align_bp=on  dbl_ovrd=off  block_type=logical
      settings: block_version=9.2.01
  Logical5 : xbsIndex_r4/Logical  logical_function=OR  inputs=2  en=off  latency=0  precision=Full  arith_type=Unsigned  n_bits=16  bin_pt=0  align_bp=on  dbl_ovrd=off  block_type=logical
      settings: block_version=9.2.01
  StRdy : xbsIndex_r4/Register  init=0  rst=off  en=off  dbl_ovrd=off  block_type=register
      settings: block_version=9.2.01
  StS : xbsIndex_r4/Register  init=0  rst=off  en=off  dbl_ovrd=off  block_type=register
      settings: block_version=9.2.01
  StSE : xbsIndex_r4/Register  init=0  rst=off  en=off  dbl_ovrd=off  block_type=register
      settings: block_version=9.2.01
  SNEn : Outport
  OVFEn : Outport  Port=2
  Rdy : Outport  Port=3
  S : Outport  Port=4
  wires:
  [NotScan] -> Logical12/2
  [Scan] -> Logical9/1
  [NotRst] -> Logical14/1
  [NotRst] -> Logical7/1
  Inverter2/1 -> [NotRst]
  [EOSAck] -> Logical2/1
  Logical12/1 -> [EOSAck]
  Inverter3/1 -> [NotScan]
  Scan/1 -> [Scan], Inverter3/1
  Logical10/1 -> Logical14/2
  Logical14/1 -> StSE/1
  [Scan] -> Logical4/2
  Logical9/1 -> Logical10/2
  StSE/1 -> Logical9/2, Logical12/1  "StSE"
  Logical5/1 -> Logical7/2
  Logical7/1 -> StS/1
  Logical6/1 -> Logical10/1, OVFEn/1
  StRdy/1 -> Rdy/1, Logical4/1, Logical/2  "Rdy"
  Logical2/1 -> StRdy/1
  StS/1 -> S/1, Logical6/1, Logical3/2  "S"
  EOS/1 -> Logical6/2, Inverter/1
  Inverter/1 -> Logical3/1
  Logical4/1 -> SNEn/1, Logical5/1
  Logical3/1 -> Logical5/2
  [NotScan] -> Logical/1
  Logical/1 -> Logical2/2
  Reset/1 -> Inverter2/1, Logical2/3

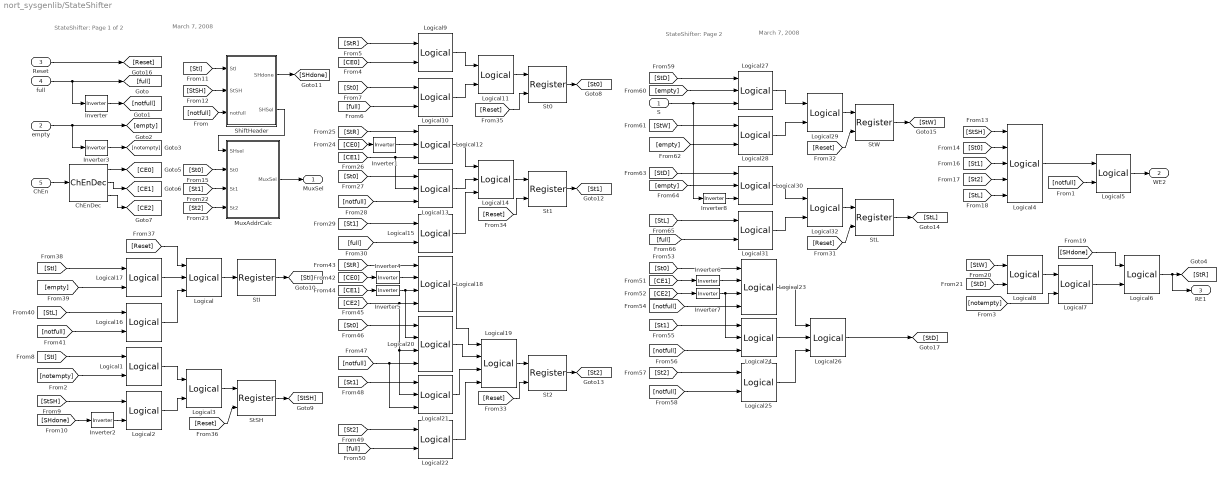
== system nort_sysgenlib/StateShifter ==
  note: March 7, 2008
  note: StateShifter: Page 2
  note: March 7, 2008
  note: StateShifter: Page 1 of 2
  S : Inport
  empty : Inport  Port=2
  Reset : Inport  Port=3
  full : Inport  Port=4
  ChEn : Inport  Port=5
  ChEnDec : nort_sysgenlib/ChEnDec  SystemSampleTime=-1
  Inverter{,1..8} (9 alike) : xbsIndex_r4/Inverter  en=off  latency=0  dbl_ovrd=off  block_type=inv
      settings: block_version=9.2.01
  Logical : xbsIndex_r4/Logical  logical_function=OR  inputs=3  en=off  latency=0  precision=Full  arith_type=Unsigned  n_bits=16  bin_pt=0  align_bp=on  dbl_ovrd=off  block_type=logical
      settings: block_version=9.2.01
  Logical{1..2,5,7,9..10,15..17,22,25,28,31} (13 alike) : xbsIndex_r4/Logical  logical_function=AND  inputs=2  en=off  latency=0  precision=Full  arith_type=Unsigned  n_bits=16  bin_pt=0  align_bp=on  dbl_ovrd=off  block_type=logical
      settings: block_version=9.2.01
  Logical{3,6,8,11,29,32} (6 alike) : xbsIndex_r4/Logical  logical_function=OR  inputs=2  en=off  latency=0  precision=Full  arith_type=Unsigned  n_bits=16  bin_pt=0  align_bp=on  dbl_ovrd=off  block_type=logical
      settings: block_version=9.2.01
  Logical{12..13,21,24,27,30} (6 alike) : xbsIndex_r4/Logical  logical_function=AND  inputs=3  en=off  latency=0  precision=Full  arith_type=Unsigned  n_bits=16  bin_pt=0  align_bp=on  dbl_ovrd=off  block_type=logical
      settings: block_version=9.2.01
  Logical14 : xbsIndex_r4/Logical  logical_function=OR  inputs=3  en=off  latency=0  precision=Full  arith_type=Unsigned  n_bits=16  bin_pt=0  align_bp=on  dbl_ovrd=off  block_type=logical
      settings: block_version=9.2.01
  Logical18 : xbsIndex_r4/Logical  logical_function=AND  inputs=4  en=off  latency=0  precision=Full  arith_type=Unsigned  n_bits=16  bin_pt=0  align_bp=on  dbl_ovrd=off  block_type=logical
      settings: block_version=9.2.01
  Logical19 : xbsIndex_r4/Logical  logical_function=OR  inputs=4  en=off  latency=0  precision=Full  arith_type=Unsigned  n_bits=16  bin_pt=0  align_bp=on  dbl_ovrd=off  block_type=logical
      settings: block_version=9.2.01
  Logical20 : xbsIndex_r4/Logical  logical_function=AND  inputs=4  en=off  latency=0  precision=Full  arith_type=Unsigned  n_bits=16  bin_pt=0  align_bp=on  dbl_ovrd=off  block_type=logical
      settings: block_version=9.2.01
  Logical23 : xbsIndex_r4/Logical  logical_function=AND  inputs=4  en=off  latency=0  precision=Full  arith_type=Unsigned  n_bits=16  bin_pt=0  align_bp=on  dbl_ovrd=off  block_type=logical
      settings: block_version=9.2.01
  Logical26 : xbsIndex_r4/Logical  logical_function=OR  inputs=3  en=off  latency=0  precision=Full  arith_type=Unsigned  n_bits=16  bin_pt=0  align_bp=on  dbl_ovrd=off  block_type=logical
      settings: block_version=9.2.01
  Logical4 : xbsIndex_r4/Logical  logical_function=OR  inputs=5  en=off  latency=0  precision=Full  arith_type=Unsigned  n_bits=16  bin_pt=0  align_bp=on  dbl_ovrd=off  block_type=logical
      settings: block_version=9.2.01
  MuxAddrCalc : Subsystem
  ShiftHeader : Subsystem
  St0 : xbsIndex_r4/Register  init=0  rst=on  en=off  dbl_ovrd=off  block_type=register
      settings: block_version=9.2.01
  St1 : xbsIndex_r4/Register  init=0  rst=on  en=off  dbl_ovrd=off  block_type=register
      settings: block_version=9.2.01
  St2 : xbsIndex_r4/Register  init=0  rst=on  en=off  dbl_ovrd=off  block_type=register
      settings: block_version=9.2.01
  StI : xbsIndex_r4/Register  init=0  rst=off  en=off  dbl_ovrd=off  block_type=register
      settings: block_version=9.2.01
  StL : xbsIndex_r4/Register  init=0  rst=on  en=off  dbl_ovrd=off  block_type=register
      settings: block_version=9.2.01
  StSH : xbsIndex_r4/Register  init=0  rst=on  en=off  dbl_ovrd=off  block_type=register
      settings: block_version=9.2.01
  StW : xbsIndex_r4/Register  init=0  rst=on  en=off  dbl_ovrd=off  block_type=register
      settings: block_version=9.2.01
  MuxSel : Outport
  WE2 : Outport  Port=2
  RE1 : Outport  Port=3
  wires:
  [notempty] -> Logical7/2
  Logical32/1 -> StL/1
  Logical31/1 -> Logical32/2
  Logical30/1 -> Logical32/1
  [full] -> Logical31/2
  [StL] -> Logical31/1
  Inverter8/1 -> Logical30/3
  [empty] -> Logical30/2
  [StD] -> Logical30/1
  Logical28/1 -> Logical29/2
  Logical27/1 -> Logical29/1
  Logical29/1 -> StW/1
  [empty] -> Logical28/2
  [StW] -> Logical28/1
  S/1 -> Inverter8/1, Logical27/3
  [empty] -> Logical27/2
  [StD] -> Logical27/1
  Logical26/1 -> [StD]
  Logical25/1 -> Logical26/3
  Logical24/1 -> Logical26/2
  Logical23/1 -> Logical26/1
  [notfull] -> Logical25/2
  [St2] -> Logical25/1
  [notfull] -> Logical24/3
  [St1] -> Logical24/1
  [notfull] -> Logical23/4
  Inverter7/1 -> Logical24/2, Logical23/3
  Inverter6/1 -> Logical23/2
  [St0] -> Logical23/1
  [CE2] -> Inverter7/1
  [CE1] -> Inverter6/1
  Logical22/1 -> Logical19/4
  Logical21/1 -> Logical19/3
  [full] -> Logical22/2
  [St2] -> Logical22/1
  [St1] -> Logical21/1
  Logical20/1 -> Logical19/2
  [notfull] -> Logical21/3, Logical20/4
  [St0] -> Logical20/1
  Logical18/1 -> Logical19/1
  Logical19/1 -> St2/1
  [CE2] -> Logical21/2, Logical20/3, Logical18/4
  Inverter5/1 -> Logical20/2, Logical18/3
  Inverter4/1 -> Logical18/2
  [CE1] -> Inverter5/1
  [StR] -> Logical18/1
  [CE0] -> Inverter4/1
  [notfull] -> Logical16/2
  [StL] -> Logical16/1
  [empty] -> Logical17/2
  [StI] -> Logical17/1
  Logical16/1 -> Logical/3
  Logical17/1 -> Logical/2
  [Reset] -> Logical/1
  [Reset] -> StSH/2
  [Reset] -> St0/2
  [Reset] -> St1/2
  [Reset] -> St2/2
  [Reset] -> StW/2
  [Reset] -> StL/2
  Reset/1 -> [Reset]
  Logical14/1 -> St1/1
  Logical15/1 -> Logical14/3
  Logical13/1 -> Logical14/2
  Logical12/1 -> Logical14/1
  [full] -> Logical15/2
  [St1] -> Logical15/1
  [notfull] -> Logical13/3
  [St0] -> Logical13/1
  [CE1] -> Logical13/2, Logical12/3
  [StR] -> Logical12/1
  Inverter1/1 -> Logical12/2
  [CE0] -> Inverter1/1
  Logical3/1 -> StSH/1
  [St2] -> MuxAddrCalc/4(St2)
  [St1] -> MuxAddrCalc/3(St1)
  [StL] -> Logical4/5
  [St2] -> Logical4/4
  [St1] -> Logical4/3
  [StW] -> Logical8/1
  StW/1 -> [StW]
  [SHdone] -> Logical6/1
  StL/1 -> [StL]
  St2/1 -> [St2]
  [St0] -> MuxAddrCalc/2(St0)
  [St0] -> Logical4/2
  [StSH] -> Logical4/1
  [StSH] -> ShiftHeader/2(StSH)
  [StI] -> ShiftHeader/1(StI)
  [SHdone] -> Inverter2/1
  [StSH] -> Logical2/1
  [StI] -> Logical1/1
  Logical11/1 -> St0/1
  Logical10/1 -> Logical11/2
  Logical9/1 -> Logical11/1
  [St0] -> Logical10/1
  [full] -> Logical10/2
  [CE0] -> Logical9/2
  [StR] -> Logical9/1
  ChEnDec/3 -> [CE2]
  ChEnDec/2 -> [CE1]
  ChEnDec/1 -> [CE0]
  Logical6/1 -> [StR], RE1/1
  [StD] -> Logical8/2
  Logical8/1 -> Logical7/1
  Logical7/1 -> Logical6/2
  [notfull] -> Logical5/2
  Inverter3/1 -> [notempty]
  empty/1 -> Inverter3/1, [empty]
  ChEn/1 -> ChEnDec/1
  Logical5/1 -> WE2/1
  Logical4/1 -> Logical5/1
  Logical2/1 -> Logical3/2
  Logical1/1 -> Logical3/1
  Inverter2/1 -> Logical2/2
  ShiftHeader/1(SHdone) -> [SHdone]
  [notempty] -> Logical1/2
  MuxAddrCalc/1(MuxSel) -> MuxSel/1
  ShiftHeader/2(SHSel) -> MuxAddrCalc/1(SHsel)
  St1/1 -> [St1]
  St0/1 -> [St0]
  Inverter/1 -> [notfull]
  [notfull] -> ShiftHeader/3(notfull)
  StSH/1 -> [StSH]
  full/1 -> Inverter/1, [full]
  StI/1 -> [StI]
  Logical/1 -> StI/1

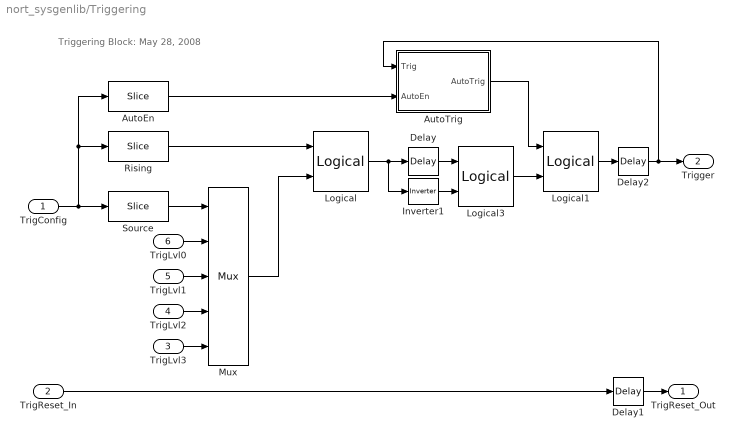
== system nort_sysgenlib/Triggering ==
  note: Triggering Block: May 28, 2008
  TrigConfig : Inport
  TrigReset_In : Inport  Port=2
  TrigLvl3 : Inport  Port=3
  TrigLvl2 : Inport  Port=4
  TrigLvl1 : Inport  Port=5
  TrigLvl0 : Inport  Port=6
  AutoEn : xbsIndex_r4/Slice  nbits=1  boolean_output=on  mode=Lower Bit Location + Width  bit1=0  base1=MSB of Input  bit0=3  base0=LSB of Input  dbl_ovrd=off  block_type=slice
      settings: infoedit="Extracts a given range of bits from each input sample and presents it at the output.  The output type is ordinarily unsigned with binary point at zero, but can be Boolean when the slice is one bit wide.<P><P>Hardware notes: In hardware this block costs nothing."  block_version=9.2.01
  AutoTrig : Subsystem
  Delay : xbsIndex_r4/Delay  en=off  latency=1  dbl_ovrd=off  reg_retiming=off  block_type=delay
      settings: block_version=9.1.01
  Delay1 : xbsIndex_r4/Delay  en=off  latency=1  dbl_ovrd=off  reg_retiming=off  block_type=delay
      settings: block_version=9.1.01
  Delay2 : xbsIndex_r4/Delay  en=off  latency=1  dbl_ovrd=off  reg_retiming=off  block_type=delay
      settings: block_version=9.1.01
  Inverter1 : xbsIndex_r4/Inverter  en=off  latency=0  dbl_ovrd=off  block_type=inv
      settings: block_version=9.1.01
  Logical : xbsIndex_r4/Logical  logical_function=XOR  inputs=2  en=off  latency=0  precision=Full  arith_type=Unsigned  n_bits=16  bin_pt=0  align_bp=on  dbl_ovrd=off  block_type=logical
      settings: block_version=9.2.01
  Logical1 : xbsIndex_r4/Logical  logical_function=OR  inputs=2  en=off  latency=0  precision=Full  arith_type=Unsigned  n_bits=16  bin_pt=0  align_bp=on  dbl_ovrd=off  block_type=logical
      settings: block_version=9.1.01
  Logical3 : xbsIndex_r4/Logical  logical_function=AND  inputs=2  en=off  latency=0  precision=Full  arith_type=Unsigned  n_bits=16  bin_pt=0  align_bp=on  dbl_ovrd=off  block_type=logical
      settings: block_version=9.1.01
  Mux : xbsIndex_r4/Mux  inputs=4  en=off  latency=0  precision=Full  arith_type=Unsigned  n_bits=16  bin_pt=14  quantization=Truncate  overflow=Wrap  dbl_ovrd=off  block_type=mux
      settings: block_version=9.2.01
  Rising : xbsIndex_r4/Slice  nbits=1  boolean_output=on  mode=Lower Bit Location + Width  bit1=0  base1=MSB of Input  bit0=2  base0=LSB of Input  dbl_ovrd=off  block_type=slice
      settings: infoedit="Extracts a given range of bits from each input sample and presents it at the output.  The output type is ordinarily unsigned with binary point at zero, but can be Boolean when the slice is one bit wide.<P><P>Hardware notes: In hardware this block costs nothing."  block_version=9.2.01
  Source : xbsIndex_r4/Slice  nbits=2  boolean_output=off  mode=Lower Bit Location + Width  bit1=0  base1=MSB of Input  bit0=0  base0=LSB of Input  dbl_ovrd=off  block_type=slice
      settings: infoedit="Extracts a given range of bits from each input sample and presents it at the output.  The output type is ordinarily unsigned with binary point at zero, but can be Boolean when the slice is one bit wide.<P><P>Hardware notes: In hardware this block costs nothing."  block_version=9.2.01
  TrigReset_Out : Outport
  Trigger : Outport  Port=2
  wires:
  Delay2/1 -> Trigger/1, AutoTrig/1(Trig)
  Delay1/1 -> TrigReset_Out/1
  TrigReset_In/1 -> Delay1/1
  TrigLvl3/1 -> Mux/5
  TrigLvl2/1 -> Mux/4
  TrigLvl1/1 -> Mux/3
  TrigLvl0/1 -> Mux/2
  Logical1/1 -> Delay2/1
  AutoTrig/1(AutoTrig) -> Logical1/1
  Logical3/1 -> Logical1/2
  AutoEn/1 -> AutoTrig/2(AutoEn)
  Inverter1/1 -> Logical3/2
  Delay/1 -> Logical3/1
  Logical/1 -> Inverter1/1, Delay/1
  Rising/1 -> Logical/1
  Mux/1 -> Logical/2
  Source/1 -> Mux/1
  TrigConfig/1 -> Source/1, Rising/1, AutoEn/1
